simulink model "powersupply_1jan_old_top"  (R2015b)
settings: Solver=ode45  StartTime=0.0  StopTime=20*T_mach  MaxStep=4e-7  MinStep=1e-8  RelTol=1e-3
values from neighbouring files (symbols this model uses):
  c2_val = (1-V_ref/Vd_val)/(8*v2_ripple*l2_val*f_sw^2)    (= 0.0001)    [PowerSupplyScript.m]    (also in master_conv.m; master_conv2.m = 6.25e-07; matlab.mat = 1e-05; normal_buck_comparison.m = 1e-05)
  Cs = (Cs_min + Cs_max) / 2    (= 1.43223295455e-05)    [PowerSupplyScript.m]    (also in QdSnubber.m = (Cs_min + Cs_max) / 2; master_conv2.m = 3.126125e-05; matlab.mat = 2.98407954545e-05)
  delay_load = t1    (= 6e-06)    [PowerSupplyScript.m]    (also in master_conv.m; master_conv2.m; matlab.mat)
  delayVC = 2e-3    (= 0.002)    [PowerSupplyScript.m]    (also in master_conv.m = 0.001; master_conv2.m = 0; matlab.mat = 0)
  den_c1 =     [matlab.mat]
  den_c2 =     [matlab.mat]
  duty_inv = 100 - duty    (= 90)    [PowerSupplyScript.m]    (also in master_conv.m; master_conv2.m; matlab.mat)
  duty_load = (t2-t1)/T_mach*100    (= 7)    [PowerSupplyScript.m]    (also in master_conv.m; master_conv2.m; matlab.mat)
  f_sw = 50e3    (= 50000)    [PowerSupplyScript.m]    (also in master_conv.m; master_conv2.m; matlab.mat)
  frq_dc = 50    [master_conv2.m]    (also in matlab.mat = 10)
  I_ref = 10    [PowerSupplyScript.m]    (also in master_conv.m; master_conv2.m; matlab.mat)
  l1_val = Vo1*(Vd_val-Vo1)/(delta_i1*f_sw*Vd_val)    (= 0.00181818181818)    [PowerSupplyScript.m]    (also in master_conv.m = 0.000181818181818; master_conv2.m; matlab.mat; poles_locus.m = l1_val_bak)
  l2_val = 2.5*r_val*(Vd_val-V_ref)/(f_sw*Vd_val)    (= 1.36363636364e-05)    [PowerSupplyScript.m]    (also in master_conv.m; master_conv2.m = 0.00218181818182; matlab.mat = 0.002; poles_locus.m = l2_val_bak)
  num_c1 =     [matlab.mat]
  num_c2 =     [matlab.mat]
  r_val = 1    [PowerSupplyScript.m]    (also in master_conv.m; master_conv2.m; matlab.mat)
  rc2_val = 0.0001    [PowerSupplyScript.m]    (also in master_conv.m; master_conv2.m; matlab.mat)
  rl1_val = 0.0002    [PowerSupplyScript.m]    (also in master_conv.m; master_conv2.m; matlab.mat)
  rl2_val = 0.0001    [PowerSupplyScript.m]    (also in master_conv.m; master_conv2.m; matlab.mat)
  Rs = V_ref / I_ref    (= 8)    [PowerSupplyScript.m]    (also in QdSnubber.m = V_ref / I_ref; master_conv2.m; matlab.mat)
  t2 = duty * T_mach / 100    (= 2e-05)    [PowerSupplyScript.m]    (also in master_conv.m; master_conv2.m; matlab.mat)
  T_mach = 200e-6    (= 0.0002)    [PowerSupplyScript.m]    (also in master_conv.m; master_conv2.m; matlab.mat)
  V_ref = 80    [PowerSupplyScript.m]    (also in master_conv.m; master_conv2.m; matlab.mat)
  Vd_val = 110    [PowerSupplyScript.m]    (also in master_conv.m; master_conv2.m; matlab.mat)
libraries: powerlib x86, simulink x10, powerlib_meascontrol x8, simulink_extras x6
(part 1 of 2)
settings Model: Creator=Akshay  LastModifiedBy=Akshay
settings SolverCC: ZeroCrossAlgorithm=Adaptive
settings DataIOCC: SaveFormat=StructureWithTime
settings HardwareCC: ProdWordSize=32  ProdHWDeviceType=Specified

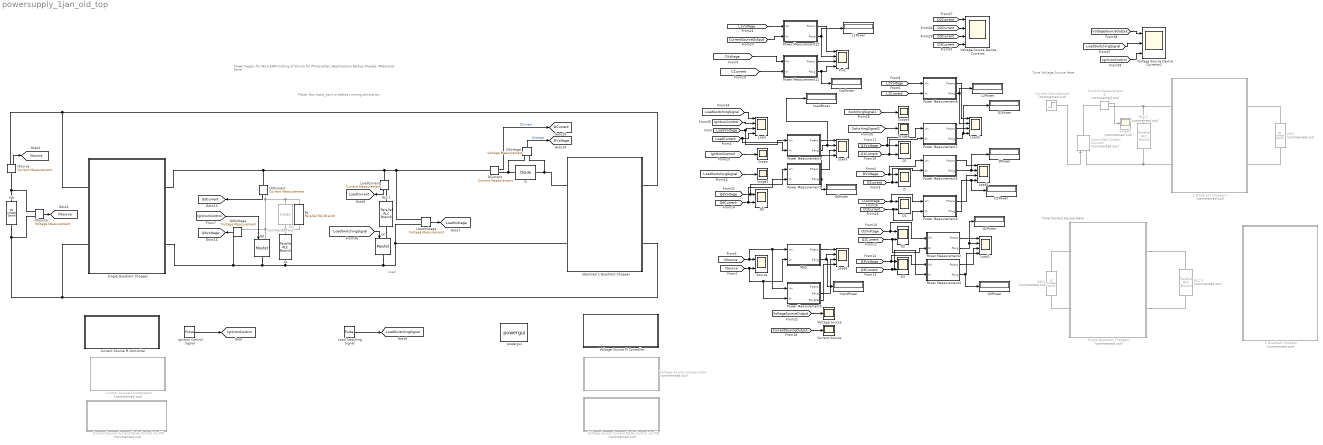
== system powersupply_1jan_old_top ==
  note: Tune Current Source Here
  note: Tune Voltage Source Here
  note: Power Supply for Wire EDM Cutting of Silicon for Photovoltaic Applications
      |
      | Akshay Khadse, Makarand Kane
  note: Load
  note: *Note: Run mast_conv.m before running simulation
  " RLC 1" : powerlib/Elements/Parallel RLC Branch  LConnTagsString=a  RConnTagsString=__new0  BranchType=R  Resistance=r_val  Inductance=1e-3  SetiL0=off  InitialCurrent=0  Capacitance=0.1e-6  Setx0=off  InitialVoltage=0  Measurements=None
  " RLC 2" : powerlib/Elements/Parallel RLC Branch  Commented=on  LConnTagsString=a  RConnTagsString=__new0  BranchType=R  Resistance=r_val  Inductance=1e-3  SetiL0=off  InitialCurrent=0  Capacitance=0.1e-6  Setx0=off  InitialVoltage=0  Measurements=None
  " RLC 3" : powerlib/Elements/Parallel RLC Branch  Commented=on  LConnTagsString=a  RConnTagsString=__new0  BranchType=R  Resistance=r_val  Inductance=1e-3  SetiL0=off  InitialCurrent=0  Capacitance=0.1e-6  Setx0=off  InitialVoltage=0  Measurements=None
  " Rs" : powerlib/Elements/Parallel RLC Branch  LConnTagsString=a  RConnTagsString=__new0  BranchType=R  Resistance=Rs  Inductance=1e-3  SetiL0=off  InitialCurrent=0  Capacitance=0.1e-6  Setx0=off  InitialVoltage=0  Measurements=None
  2 Quadrant Chopper : Subsystem  Commented=on
  2 Quadrant Chopper1 : Subsystem  Commented=on
  CapPower : Display
  Controlled Current Source1 : powerlib/Electrical Sources/Controlled Current Source  Commented=on  Initialize=on  Source_Type=AC  Amplitude=0  Phase=0  Frequency=0  Measurements=None
  Cs : powerlib/Elements/Parallel RLC Branch  LConnTagsString=a  RConnTagsString=__new0  BranchType=C  Resistance=r_val  Inductance=1e-3  SetiL0=off  InitialCurrent=0  Capacitance=Cs  Setx0=off  InitialVoltage=0  Measurements=None
  Current Disturbance1 : Step  Commented=on  Time=1e-3  After=10  SampleTime=0
  Current Measurement3 : powerlib/Measurements/Current Measurement  Commented=on  PhasorSimulation=off  OutputType=Complex  PSBequivalent=0
  Current Source : Scope
  Current Source Compensator : Subsystem  Commented=on
  Current Source Current Mode Control via PID : Subsystem  Commented=on
  Current Source PI Controller : Subsystem
  D : powerlib/Power Electronics/Diode  Ron=0.001  Lon=0  Vf=0.8  IC=0  UseSnubber=off  Rs=500  Cs=250e-9  Measurements=off
  "D " : Scope  NumInputPorts=2
  D1 : Scope  NumInputPorts=2
  D1Power : Display
  DCurrent : powerlib/Measurements/Current Measurement  PhasorSimulation=off  OutputType=Complex  PSBequivalent=0
  DPower : Display
  DVoltage : powerlib/Measurements/Voltage Measurement  PhasorSimulation=off  OutputType=Complex  PSBequivalent=0
  Ds : powerlib/Power Electronics/Diode  Commented=on  Ron=0.001  Lon=0  Vf=0.8  IC=0  UseSnubber=off  Rs=500  Cs=250e-9  Measurements=off
  ISource : powerlib/Measurements/Current Measurement  PhasorSimulation=off  OutputType=Complex  PSBequivalent=0
  Idealized 2 Quadrant Chopper : Subsystem
  Ignition Control Signal : DiscretePulseGenerator  PulseType=Time based  Period=T_mach  PulseWidth=duty_inv  PhaseDelay=t2 + delayVC
  InputPower : Display
  L1Power : Display
  L2Power : Display
  Load{,1..3,5..6} (6 alike) : Scope  NumInputPorts=4
  Load Switching Signal : DiscretePulseGenerator  PulseType=Time based  Period=T_mach  PulseWidth=duty_load  PhaseDelay=delay_load + delayVC
  LoadCurrent : powerlib/Measurements/Current Measurement  PhasorSimulation=off  OutputType=Complex  PSBequivalent=0
  LoadPower : Display
  LoadVoltage : powerlib/Measurements/Voltage Measurement  PhasorSimulation=off  OutputType=Complex  PSBequivalent=0
  PM0 : Subsystem
  Pm1 : Scope  NumInputPorts=4
  Power Measurement1 : Subsystem
  Power Measurement11 : Subsystem
  Power Measurement12 : Subsystem
  Power Measurement2 : Subsystem
  Power Measurement3 : Subsystem
  Power Measurement4 : Subsystem
  Power Measurement5 : Subsystem
  Power Measurement6 : Subsystem
  Power Measurement7 : Subsystem
  Power Measurement8 : Subsystem
  Power Measurement9 : Subsystem
  "Q1 " : Scope  NumInputPorts=2
  Q1Power : Display
  "Q2 " : Scope  NumInputPorts=2
  Q2Power : Display
  "Q3 " : Scope  NumInputPorts=2
  Q3Power : Display
  Qd : powerlib/Power Electronics/Mosfet  Ron=0.1  Lon=0  Rd=0.01  Vfd=0  IC=0  Rs=1e5  Cs=inf  Measurements=off
  "Qd " : Scope  NumInputPorts=2
  QdCurrent : powerlib/Measurements/Current Measurement  PhasorSimulation=off  OutputType=Complex  PSBequivalent=0
  QdPower : Display
  QdVoltage : powerlib/Measurements/Voltage Measurement  PhasorSimulation=off  OutputType=Complex  PSBequivalent=0
  Ql : powerlib/Power Electronics/Mosfet  Ron=0.1  Lon=0  Rd=0.01  Vfd=0  IC=0  Rs=1e5  Cs=inf  Measurements=off
  Scope{,1,5..6} (4 alike) : Scope
  Scope2 : Scope  Commented=on
  Single Quadrant Chopper : Subsystem
  Single Quadrant Chopper1 : Subsystem  Commented=on
  Source : Scope  NumInputPorts=2
  VSource : powerlib/Measurements/Voltage Measurement  PhasorSimulation=off  OutputType=Complex  PSBequivalent=0
  Vdc : powerlib/Electrical Sources/DC Voltage Source  Amplitude=Vd_val  Measurements=Voltage
  Vdc1 : powerlib/Electrical Sources/DC Voltage Source  Commented=on  Amplitude=Vd_val  Measurements=Voltage
  Vdc2 : powerlib/Electrical Sources/DC Voltage Source  Commented=on  Amplitude=Vd_val  Measurements=Voltage
  Voltage Source : Scope
  Voltage Source Device Currents : Scope  NumInputPorts=4
  Voltage Source Device Currents1 : Scope  NumInputPorts=3
  Voltage Source Compensator : Subsystem  Commented=on
  Voltage Source Current Mode Control via PID : Subsystem  Commented=on
  Voltage Source PI Controller : Subsystem
  powergui : powerlib/powergui  Priority=1  SimulationMode=Discrete  SolverType=Backward Euler  SampleTime=0.01/f_sw  frequency=60  SPID=on  DisableSnubberDevices=off  DisableRonSwitches=off  DisableVfSwitches=off  SwTol=0  DisplayEquations=off  Interpol=off  ExternalGateDelay=off  methode=off  Ts=0  FunctionMessages=off  echomessages=off  HookPort=off  EnableUseOfTLC=off  x0status=zero  frequencyindice=0  Pbase=100e6  ErrMax=1e-4  Iterations=50  UnitsV=kV  UnitsW=MW  buscounter=0  RestoreLinks=warning  ResistiveCurrentMeasurement=off  Frange=[0:2:500]  Ylog=off  Xlog=on  ShowGrid=off  save=off  variable=ZData  structure=ScopeData  ZoomFFT=off  StartTime=0.0  cycles=5  DisplayStyle=2  fundamental=50  FreqAxis=off  MaxFrequency=50000  frequencyindicesteady=1  RmsSteady=1  display=off
  tag scope: DCurrent=global, DVoltage=global, ISource=global, IgnitionControl=global, LoadCurrent=global, LoadSwitchingSignal=global, LoadVoltage=global, QdCurrent=global, QdVoltage=global, VSource=global
  wires:
  Ignition Control Signal/1 -> [IgnitionControl]
  Load Switching Signal/1 -> [LoadSwitchingSignal]
  [Q2Voltage] -> Power Measurement2/1(Vin), "Q2 "/1
  [Q2Current] -> Power Measurement2/2(Iin), "Q2 "/2
  [Q3Voltage] -> Power Measurement4/1(Vin), "Q3 "/1
  [Q3Current] -> Power Measurement4/2(Iin), "Q3 "/2
  [Q1Voltage] -> Power Measurement7/1(Vin), "Q1 "/1
  [Q1Current] -> Power Measurement7/2(Iin), "Q1 "/2
  [QdVoltage] -> Power Measurement1/1(Vin), "Qd "/1
  [QdCurrent] -> Power Measurement1/2(Iin), "Qd "/2
  [IgnitionControl] -> Scope/1
  [LoadSwitchingSignal] -> Scope1/1
  LoadCurrent/1 -> [LoadCurrent]
  LoadVoltage/1 -> [LoadVoltage]
  [IgnitionControl] -> Qd/1
  QdCurrent/1 -> [QdCurrent]
  QdVoltage/1 -> [QdVoltage]
  DVoltage/1 -> [DVoltage]  "DVoltage"
  DCurrent/1 -> [DCurrent]  "DCurrent"
  [LoadSwitchingSignal] -> Load/1
  [IgnitionControl] -> Load/2
  [LoadVoltage] -> Power Measurement9/1(Vin), Load/3
  [LoadCurrent] -> Power Measurement9/2(Iin), Load/4
  [LoadSwitchingSignal] -> Ql/1
  [SwitchingSignal2] -> Scope6/1
  [SwitchingSignal1] -> Scope5/1
  [DVoltage] -> Power Measurement5/1(Vin), "D "/1
  [DCurrent] -> Power Measurement5/2(Iin), "D "/2
  VSource/1 -> [VSource]
  ISource/1 -> [ISource]
  [VSource] -> Power Measurement3/1(Vin), PM0/1(Vin), Source/1
  [ISource] -> Power Measurement3/2(Iin), PM0/2(Iin), Source/2
  [D1Voltage] -> Power Measurement6/1(Vin), D1/1
  Current Disturbance1/1 -> Controlled Current Source1/1
  Current Measurement3/1 -> Scope2/1
  Power Measurement2/1(Ptrans) -> Load1/1
  Power Measurement2/2(Pavg) -> Load1/2, Q2Power/1
  Power Measurement4/1(Ptrans) -> Load1/3
  Power Measurement4/2(Pavg) -> Load1/4, Q3Power/1
  [D1Current] -> Power Measurement6/2(Iin), D1/2
  Power Measurement5/1(Ptrans) -> Load5/1
  Power Measurement5/2(Pavg) -> Load5/2, DPower/1
  Power Measurement6/1(Ptrans) -> Load5/3
  Power Measurement6/2(Pavg) -> Load5/4, D1Power/1
  Power Measurement9/1(Ptrans) -> Load3/1
  Power Measurement9/2(Pavg) -> Load3/2, LoadPower/1
  Power Measurement1/1(Ptrans) -> Load3/3
  Power Measurement1/2(Pavg) -> Load3/4, QdPower/1
  PM0/1(Ptrans) -> Load6/1
  PM0/2(Pavg) -> Load6/2, InputPower/1
  [L2Current] -> Power Measurement8/2(Iin)
  [L2Voltage] -> Power Measurement8/1(Vin)
  Power Measurement7/2(Pavg) -> Load2/4, Q1Power/1
  Power Measurement7/1(Ptrans) -> Load2/3
  Power Measurement8/1(Ptrans) -> Load2/1
  Power Measurement8/2(Pavg) -> Load2/2, L2Power/1
  [CVoltage] -> Power Measurement11/1(Vin)
  [CCurrent] -> Power Measurement11/2(Iin)
  Power Measurement11/1(Ptrans) -> Pm1/3
  Power Measurement11/2(Pavg) -> CapPower/1, Pm1/4
  [L1Voltage] -> Power Measurement12/1(Vin)
  [CurrentSourceOutput] -> Power Measurement12/2(Iin)
  Power Measurement12/1(Ptrans) -> Pm1/1
  Power Measurement12/2(Pavg) -> L1Power/1, Pm1/2
  [VoltageSourceOutput] -> Voltage Source/1
  [CurrentSourceOutput] -> Current Source/1
  Power Measurement3/2(Pavg) -> Load6/3
  Power Measurement3/3(PavgFB) -> Load6/4
  [Q2Current] -> Voltage Source Device Currents/1
  [Q3Current] -> Voltage Source Device Currents/3
  [D3Current] -> Voltage Source Device Currents/4
  [D2Current] -> Voltage Source Device Currents/2
  [VoltageSourceOutput] -> Voltage Source Device Currents1/1
  [LoadSwitchingSignal] -> Voltage Source Device Currents1/2
  [IgnitionControl] -> Voltage Source Device Currents1/3
  connections:
  LoadCurrent/RConn1 -- " RLC 1"/LConn1
  Ds/LConn1 -- QdVoltage/LConn2 -- Qd/LConn1 -- QdCurrent/RConn1 -- " Rs"/LConn1
  DVoltage/LConn1 -- DCurrent/RConn1 -- D/LConn1
  DCurrent/LConn1 -- LoadVoltage/LConn1 -- Single Quadrant Chopper/RConn1 -- QdCurrent/LConn1 -- LoadCurrent/LConn1
  Idealized 2 Quadrant Chopper/RConn1 -- ISource/RConn1 -- Single Quadrant Chopper/LConn1
  Idealized 2 Quadrant Chopper/RConn2 -- VSource/LConn2 -- Vdc/LConn1 -- Single Quadrant Chopper/LConn2
  Ql/LConn1 -- " RLC 1"/RConn1
  Qd/RConn1 -- Idealized 2 Quadrant Chopper/LConn2 -- LoadVoltage/LConn2 -- Ql/RConn1 -- Cs/RConn1 -- Single Quadrant Chopper/RConn2 -- QdVoltage/LConn1
  ISource/LConn1 -- Vdc/RConn1 -- VSource/LConn1
  " RLC 2"/LConn1 -- Current Measurement3/RConn1 -- 2 Quadrant Chopper1/LConn1
  " RLC 2"/RConn1 -- Controlled Current Source1/LConn1 -- 2 Quadrant Chopper1/LConn2
  Vdc1/RConn1 -- 2 Quadrant Chopper1/RConn1
  Vdc1/LConn1 -- 2 Quadrant Chopper1/RConn2
  Vdc2/RConn1 -- Single Quadrant Chopper1/LConn1
  Vdc2/LConn1 -- Single Quadrant Chopper1/LConn2
  Single Quadrant Chopper1/RConn1 -- " RLC 3"/LConn1
  Single Quadrant Chopper1/RConn2 -- " RLC 3"/RConn1
  Ds/RConn1 -- " Rs"/RConn1 -- Cs/LConn1
  Controlled Current Source1/RConn1 -- Current Measurement3/LConn1
  Idealized 2 Quadrant Chopper/LConn1 -- DVoltage/LConn2 -- D/RConn1

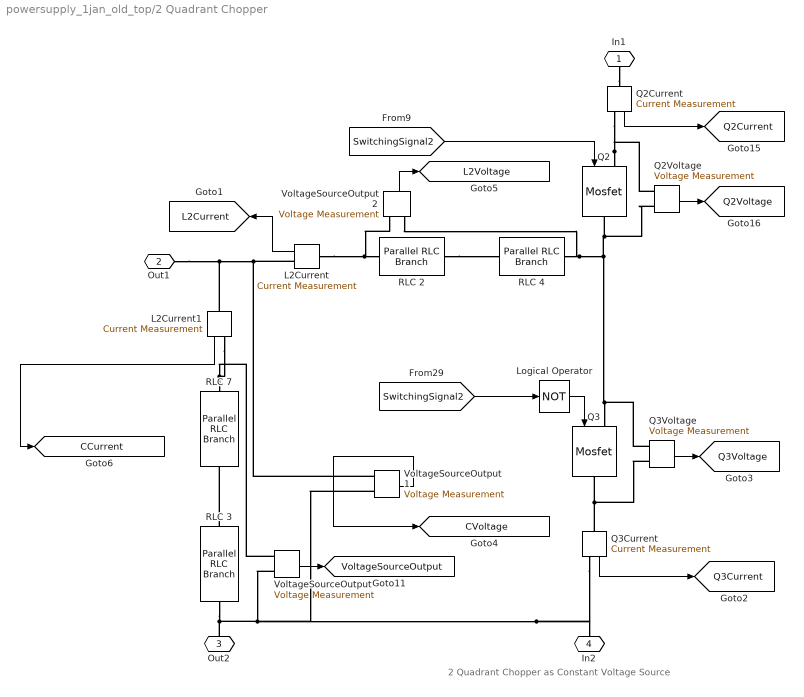
== system powersupply_1jan_old_top/2 Quadrant Chopper ==
  note: 2 Quadrant Chopper as Constant Voltage Source
  " RLC 2" : powerlib/Elements/Parallel RLC Branch  LConnTagsString=a  RConnTagsString=__new0  BranchType=R  Resistance=rl2_val  Inductance=5e-6  SetiL0=off  InitialCurrent=0  Capacitance=0.3e-6  Setx0=off  InitialVoltage=0  Measurements=None
  " RLC 3" : powerlib/Elements/Parallel RLC Branch  LConnTagsString=a  RConnTagsString=__new0  BranchType=C  Resistance=1  Inductance=1e-3  SetiL0=off  InitialCurrent=0  Capacitance=c2_val  Setx0=off  InitialVoltage=50  Measurements=None
  " RLC 4" : powerlib/Elements/Parallel RLC Branch  LConnTagsString=a  RConnTagsString=__new0  BranchType=L  Resistance=50  Inductance=l2_val  SetiL0=off  InitialCurrent=0  Capacitance=0.3e-6  Setx0=off  InitialVoltage=0  Measurements=None
  " RLC 7" : powerlib/Elements/Parallel RLC Branch  LConnTagsString=a  RConnTagsString=__new0  BranchType=R  Resistance=rc2_val  Inductance=1e-3  SetiL0=off  InitialCurrent=0  Capacitance=0.1e-6  Setx0=off  InitialVoltage=0  Measurements=None
  L2Current : powerlib/Measurements/Current Measurement  PhasorSimulation=off  OutputType=Complex  PSBequivalent=0
  L2Current1 : powerlib/Measurements/Current Measurement  PhasorSimulation=off  OutputType=Complex  PSBequivalent=0
  Logical Operator : Logic  Operator=NOT  AllPortsSameDT=off  OutDataTypeStr=boolean
  Q2 : powerlib/Power Electronics/Mosfet  Ron=0.1  Lon=0  Rd=0.01  Vfd=0  IC=0  Rs=1e5  Cs=inf  Measurements=off
  Q2Current : powerlib/Measurements/Current Measurement  PhasorSimulation=off  OutputType=Complex  PSBequivalent=0
  Q2Voltage : powerlib/Measurements/Voltage Measurement  PhasorSimulation=off  OutputType=Complex  PSBequivalent=0
  Q3 : powerlib/Power Electronics/Mosfet  Ron=0.1  Lon=0  Rd=0.01  Vfd=0  IC=0  Rs=1e5  Cs=inf  Measurements=off
  Q3Current : powerlib/Measurements/Current Measurement  PhasorSimulation=off  OutputType=Complex  PSBequivalent=0
  Q3Voltage : powerlib/Measurements/Voltage Measurement  PhasorSimulation=off  OutputType=Complex  PSBequivalent=0
  VoltageSourceOutput : powerlib/Measurements/Voltage Measurement  PhasorSimulation=off  OutputType=Complex  PSBequivalent=0
  VoltageSourceOutput1 : powerlib/Measurements/Voltage Measurement  PhasorSimulation=off  OutputType=Complex  PSBequivalent=0
  VoltageSourceOutput2 : powerlib/Measurements/Voltage Measurement  PhasorSimulation=off  OutputType=Complex  PSBequivalent=0
  In1 : PMIOPort  Port=1  Side=Right
  Out1 : PMIOPort  Port=2  Side=Left
  Out2 : PMIOPort  Port=3  Side=Left
  In2 : PMIOPort  Port=4  Side=Right
  tag scope: CCurrent=global, CVoltage=global, L2Current=global, L2Voltage=global, Q2Current=global, Q2Voltage=global, Q3Current=global, Q3Voltage=global, VoltageSourceOutput=global
  wires:
  Logical Operator/1 -> Q3/1
  VoltageSourceOutput/1 -> [VoltageSourceOutput]
  Q3Current/1 -> [Q3Current]
  Q3Voltage/1 -> [Q3Voltage]
  Q2Voltage/1 -> [Q2Voltage]
  Q2Current/1 -> [Q2Current]
  [SwitchingSignal2] -> Q2/1
  [SwitchingSignal2] -> Logical Operator/1
  L2Current/1 -> [L2Current]
  VoltageSourceOutput1/1 -> [CVoltage]
  VoltageSourceOutput2/1 -> [L2Voltage]
  L2Current1/1 -> [CCurrent]
  connections:
  " RLC 3"/RConn1 -- VoltageSourceOutput1/LConn2 -- Q3Current/RConn1 -- In2/RConn1 -- VoltageSourceOutput/LConn2 -- Out2/RConn1
  " RLC 3"/LConn1 -- " RLC 7"/RConn1
  Q3Voltage/LConn2 -- Q3Current/LConn1 -- Q3/RConn1
  Q2/LConn1 -- Q2Voltage/LConn1 -- Q2Current/RConn1
  " RLC 2"/RConn1 -- " RLC 4"/LConn1
  In1/RConn1 -- Q2Current/LConn1
  Out1/RConn1 -- L2Current1/LConn1 -- VoltageSourceOutput1/LConn1 -- L2Current/RConn1
  " RLC 4"/RConn1 -- Q3Voltage/LConn1 -- Q3/LConn1 -- Q2Voltage/LConn2 -- Q2/RConn1 -- VoltageSourceOutput2/LConn2
  L2Current/LConn1 -- VoltageSourceOutput2/LConn1 -- " RLC 2"/LConn1
  " RLC 7"/LConn1 -- L2Current1/RConn1 -- VoltageSourceOutput/LConn1

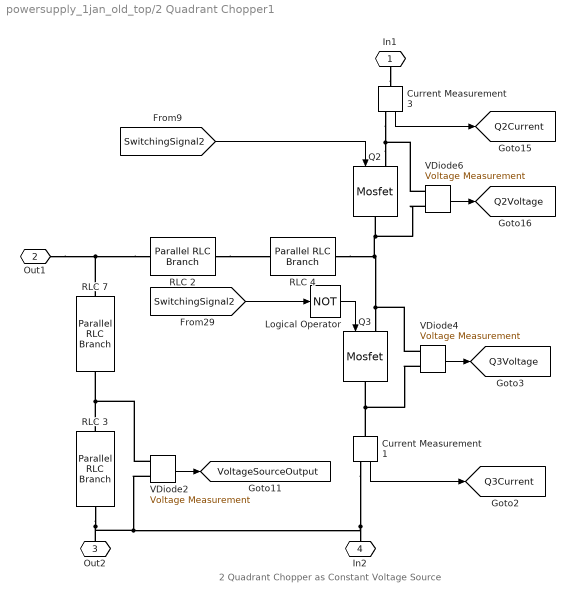
== system powersupply_1jan_old_top/2 Quadrant Chopper1 ==
  note: 2 Quadrant Chopper as Constant Voltage Source
  " RLC 2" : powerlib/Elements/Parallel RLC Branch  LConnTagsString=a  RConnTagsString=__new0  BranchType=R  Resistance=rl2_val  Inductance=5e-6  SetiL0=off  InitialCurrent=0  Capacitance=0.3e-6  Setx0=off  InitialVoltage=0  Measurements=None
  " RLC 3" : powerlib/Elements/Parallel RLC Branch  LConnTagsString=a  RConnTagsString=__new0  BranchType=C  Resistance=1  Inductance=1e-3  SetiL0=off  InitialCurrent=0  Capacitance=c2_val  Setx0=off  InitialVoltage=50  Measurements=None
  " RLC 4" : powerlib/Elements/Parallel RLC Branch  LConnTagsString=a  RConnTagsString=__new0  BranchType=L  Resistance=50  Inductance=l2_val  SetiL0=off  InitialCurrent=0  Capacitance=0.3e-6  Setx0=off  InitialVoltage=0  Measurements=None
  " RLC 7" : powerlib/Elements/Parallel RLC Branch  LConnTagsString=a  RConnTagsString=__new0  BranchType=R  Resistance=rc2_val  Inductance=1e-3  SetiL0=off  InitialCurrent=0  Capacitance=0.1e-6  Setx0=off  InitialVoltage=0  Measurements=None
  Current Measurement1 : powerlib/Measurements/Current Measurement  PhasorSimulation=off  OutputType=Complex  PSBequivalent=0
  Current Measurement3 : powerlib/Measurements/Current Measurement  PhasorSimulation=off  OutputType=Complex  PSBequivalent=0
  Logical Operator : Logic  Operator=NOT  AllPortsSameDT=off  OutDataTypeStr=boolean
  Q2 : powerlib/Power Electronics/Mosfet  Ron=0.1  Lon=0  Rd=0.01  Vfd=0  IC=0  Rs=1e5  Cs=inf  Measurements=off
  Q3 : powerlib/Power Electronics/Mosfet  Ron=0.1  Lon=0  Rd=0.01  Vfd=0  IC=0  Rs=1e5  Cs=inf  Measurements=off
  VDiode2 : powerlib/Measurements/Voltage Measurement  PhasorSimulation=off  OutputType=Complex  PSBequivalent=0
  VDiode4 : powerlib/Measurements/Voltage Measurement  PhasorSimulation=off  OutputType=Complex  PSBequivalent=0
  VDiode6 : powerlib/Measurements/Voltage Measurement  PhasorSimulation=off  OutputType=Complex  PSBequivalent=0
  In1 : PMIOPort  Port=1  Side=Right
  Out1 : PMIOPort  Port=2  Side=Left
  Out2 : PMIOPort  Port=3  Side=Left
  In2 : PMIOPort  Port=4  Side=Right
  tag scope: Q2Current=global, Q2Voltage=global, Q3Current=global, Q3Voltage=global, VoltageSourceOutput=global
  wires:
  Logical Operator/1 -> Q3/1
  VDiode2/1 -> [VoltageSourceOutput]
  Current Measurement1/1 -> [Q3Current]
  VDiode4/1 -> [Q3Voltage]
  VDiode6/1 -> [Q2Voltage]
  Current Measurement3/1 -> [Q2Current]
  [SwitchingSignal2] -> Q2/1
  [SwitchingSignal2] -> Logical Operator/1
  connections:
  " RLC 3"/RConn1 -- Current Measurement1/RConn1 -- In2/RConn1 -- VDiode2/LConn2 -- Out2/RConn1
  VDiode2/LConn1 -- " RLC 3"/LConn1 -- " RLC 7"/RConn1
  VDiode4/LConn2 -- Current Measurement1/LConn1 -- Q3/RConn1
  Q2/LConn1 -- VDiode6/LConn1 -- Current Measurement3/RConn1
  " RLC 2"/RConn1 -- " RLC 4"/LConn1
  In1/RConn1 -- Current Measurement3/LConn1
  " RLC 2"/LConn1 -- " RLC 7"/LConn1 -- Out1/RConn1
  " RLC 4"/RConn1 -- VDiode4/LConn1 -- Q3/LConn1 -- VDiode6/LConn2 -- Q2/RConn1

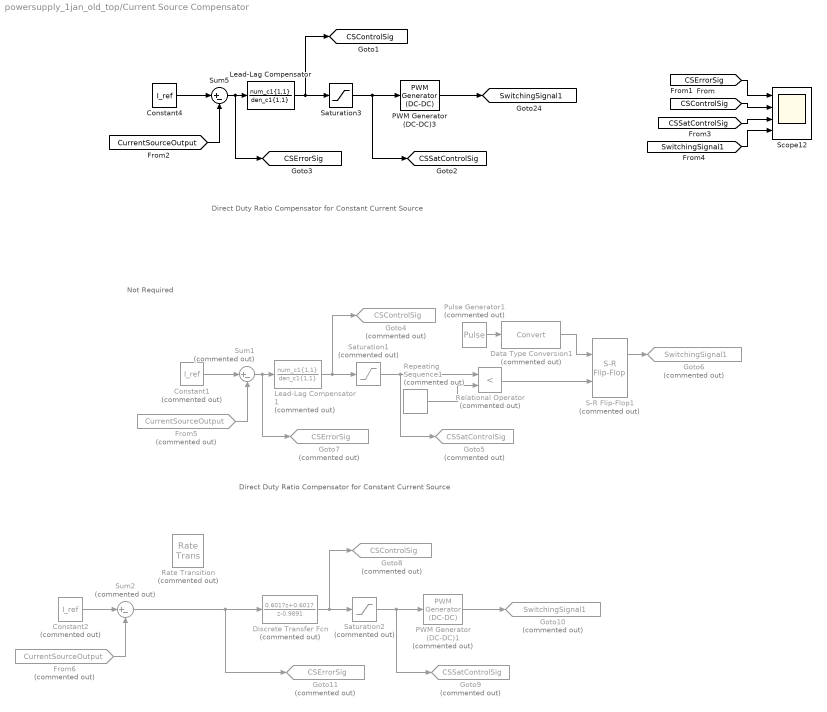
== system powersupply_1jan_old_top/Current Source Compensator ==
  note: Not Required
  note: Direct Duty Ratio Compensator for Constant Current Source
  note: Direct Duty Ratio Compensator for Constant Current Source
  Constant1 : Constant  Commented=on  Value=I_ref
  Constant2 : Constant  Commented=on  Value=I_ref
  Constant4 : Constant  Value=I_ref
  Data Type Conversion1 : DataTypeConversion  Commented=on
  Discrete Transfer Fcn : DiscreteTransferFcn  Commented=on  Numerator=[0.6017 0.6017]  Denominator=[1 -0.9891]
  From5 : From  Commented=on  GotoTag=CurrentSourceOutput  TagVisibility=global
  From6 : From  Commented=on  GotoTag=CurrentSourceOutput  TagVisibility=global
  Goto10 : Goto  Commented=on  GotoTag=SwitchingSignal1  TagVisibility=global
  Goto11 : Goto  Commented=on  GotoTag=CSErrorSig  TagVisibility=global
  Goto4 : Goto  Commented=on  GotoTag=CSControlSig  TagVisibility=global
  Goto5 : Goto  Commented=on  GotoTag=CSSatControlSig  TagVisibility=global
  Goto6 : Goto  Commented=on  GotoTag=SwitchingSignal1  TagVisibility=global
  Goto7 : Goto  Commented=on  GotoTag=CSErrorSig  TagVisibility=global
  Goto8 : Goto  Commented=on  GotoTag=CSControlSig  TagVisibility=global
  Goto9 : Goto  Commented=on  GotoTag=CSSatControlSig  TagVisibility=global
  Lead-Lag Compensator : TransferFcn  Numerator=num_c1{1,1}  Denominator=den_c1{1,1}
  Lead-Lag Compensator1 : TransferFcn  Commented=on  Numerator=num_c1{1,1}  Denominator=den_c1{1,1}
  PWM Generator (DC-DC)1 : powerlib_meascontrol/Pulse & Signal Generators/PWM Generator (DC-DC)  Commented=on  Fsw=f_sw  Ts=0
  PWM Generator (DC-DC)3 : powerlib_meascontrol/Pulse & Signal Generators/PWM Generator (DC-DC)  Fsw=f_sw  Ts=0
  Pulse Generator1 : DiscretePulseGenerator  Commented=on  PulseType=Time based  Period=1/f_sw  PulseWidth=5
  Rate Transition : RateTransition  Commented=on  OutPortSampleTime=0.01/f_sw
  Relational Operator : RelationalOperator  Commented=on  Operator=<  OutDataTypeStr=boolean
  Repeating Sequence1 : simulink/Sources/Repeating Sequence  Commented=on  rep_seq_t=[0 1/f_sw]  rep_seq_y=[0 1]
  S-R Flip-Flop1 : simulink_extras/Flip Flops/S-R Flip-Flop  Commented=on  initial_condition=0
  Saturation1 : Saturate  Commented=on  UpperLimit=0.99  LowerLimit=0
  Saturation2 : Saturate  Commented=on  UpperLimit=0.99  LowerLimit=0
  Saturation3 : Saturate  UpperLimit=0.99  LowerLimit=0
  Scope12 : Scope  NumInputPorts=4
  Sum1 : Sum  Commented=on  Inputs=|+-
  Sum2 : Sum  Commented=on  Inputs=|+-
  Sum5 : Sum  Inputs=|+-
  tag scope: CSControlSig=global, CSErrorSig=global, CSSatControlSig=global, SwitchingSignal1=global
  wires:
  Sum5/1 -> [CSErrorSig], Lead-Lag Compensator/1
  Constant4/1 -> Sum5/1
  [CurrentSourceOutput] -> Sum5/2
  Lead-Lag Compensator/1 -> Saturation3/1, [CSControlSig]
  Saturation3/1 -> [CSSatControlSig], PWM Generator (DC-DC)3/1
  PWM Generator (DC-DC)3/1 -> [SwitchingSignal1]
  [CSErrorSig] -> Scope12/1
  [CSControlSig] -> Scope12/2
  [CSSatControlSig] -> Scope12/3
  [SwitchingSignal1] -> Scope12/4
  Sum1/1 -> Goto7/1, Lead-Lag Compensator1/1
  Constant1/1 -> Sum1/1
  From5/1 -> Sum1/2
  Lead-Lag Compensator1/1 -> Saturation1/1, Goto4/1
  Saturation1/1 -> Relational Operator/1, Goto5/1
  Repeating Sequence1/1 -> Relational Operator/2
  S-R Flip-Flop1/1 -> Goto6/1
  Pulse Generator1/1 -> Data Type Conversion1/1
  Data Type Conversion1/1 -> S-R Flip-Flop1/1
  Relational Operator/1 -> S-R Flip-Flop1/2
  Constant2/1 -> Sum2/1
  From6/1 -> Sum2/2
  Discrete Transfer Fcn/1 -> Goto8/1, Saturation2/1
  Saturation2/1 -> Goto9/1, PWM Generator (DC-DC)1/1
  PWM Generator (DC-DC)1/1 -> Goto10/1
  Sum2/1 -> Goto11/1, Discrete Transfer Fcn/1

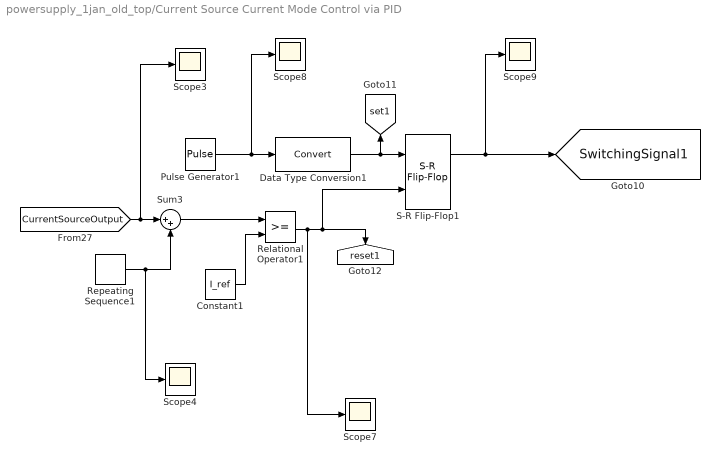
== system powersupply_1jan_old_top/Current Source Current Mode Control via PID ==
  Constant1 : Constant  Value=I_ref
  Data Type Conversion1 : DataTypeConversion
  Pulse Generator1 : DiscretePulseGenerator  PulseType=Time based  Period=1/f_sw  PulseWidth=5
  Relational Operator1 : RelationalOperator  OutDataTypeStr=boolean
  Repeating Sequence1 : simulink/Sources/Repeating Sequence  rep_seq_t=[0 1/f_sw]  rep_seq_y=[0 0]
  S-R Flip-Flop1 : simulink_extras/Flip Flops/S-R Flip-Flop  initial_condition=0
  Scope{3..4,7..9} (5 alike) : Scope
  Sum3 : Sum  Inputs=|++
  tag scope: SwitchingSignal1=global, reset1=global, set1=global
  wires:
  Pulse Generator1/1 -> Scope8/1, Data Type Conversion1/1
  Data Type Conversion1/1 -> S-R Flip-Flop1/1, [set1]
  Relational Operator1/1 -> Scope7/1, S-R Flip-Flop1/2, [reset1]
  S-R Flip-Flop1/1 -> Scope9/1, [SwitchingSignal1]
  [CurrentSourceOutput] -> Scope3/1, Sum3/1
  Repeating Sequence1/1 -> Scope4/1, Sum3/2
  Sum3/1 -> Relational Operator1/1
  Constant1/1 -> Relational Operator1/2

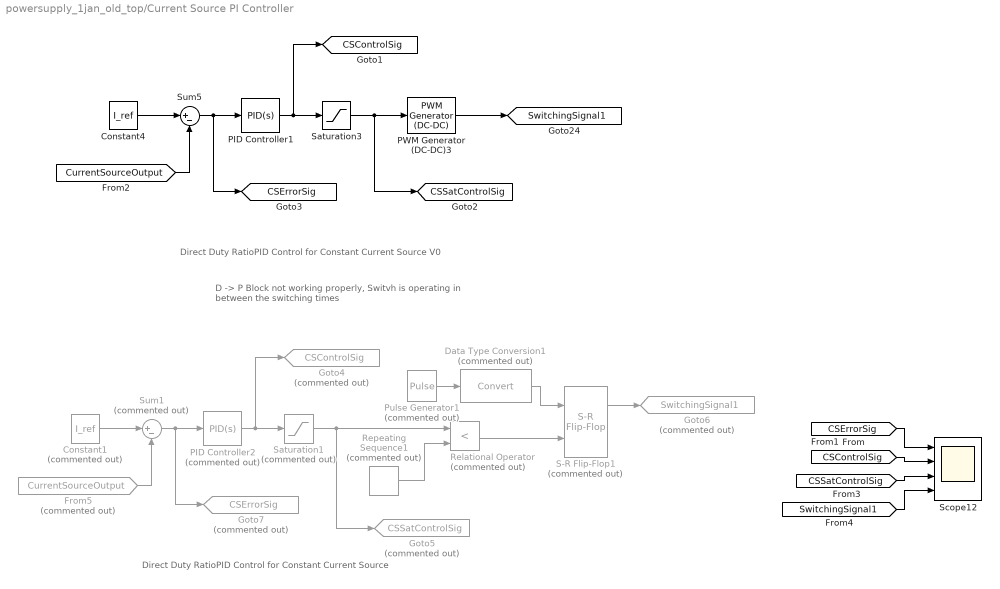
== system powersupply_1jan_old_top/Current Source PI Controller ==
  note: D -> P Block not working properly,
      | Switvh is operating in between the switching times
  note: Direct Duty RatioPID Control for Constant Current Source V0
  note: Direct Duty RatioPID Control for Constant Current Source
  Constant1 : Constant  Commented=on  Value=I_ref
  Constant4 : Constant  Value=I_ref
  Data Type Conversion1 : DataTypeConversion  Commented=on
  From5 : From  Commented=on  GotoTag=CurrentSourceOutput  TagVisibility=global
  Goto4 : Goto  Commented=on  GotoTag=CSControlSig  TagVisibility=global
  Goto5 : Goto  Commented=on  GotoTag=CSSatControlSig  TagVisibility=global
  Goto6 : Goto  Commented=on  GotoTag=SwitchingSignal1  TagVisibility=global
  Goto7 : Goto  Commented=on  GotoTag=CSErrorSig  TagVisibility=global
  PID Controller1 : simulink/Continuous/PID Controller  Controller=PID  TimeDomain=Continuous-time  SampleTime=-1  IntegratorMethod=Forward Euler  FilterMethod=Forward Euler  Form=Parallel  UseFilter=on  ControllerParametersSource=internal  P=3  I=0  D=0  N=5  InitialConditionSource=internal  InitialConditionForIntegrator=0  InitialConditionForFilter=0  ExternalReset=none  LimitOutput=off  UpperSaturationLimit=inf  LowerSaturationLimit=-inf  LinearizeAsGain=on  AntiWindupMode=none  Kb=1  TrackingMode=off  Kt=1  PParamMin=[]  PParamMax=[]  IParamMin=[]  IParamMax=[]  DParamMin=[]  DParamMax=[]  NParamMin=[]  NParamMax=[]  KbParamMin=[]  KbParamMax=[]  KtParamMin=[]  KtParamMax=[]  POutMin=[]  POutMax=[]  IOutMin=[]  IOutMax=[]  DOutMin=[]  DOutMax=[]  NOutMin=[]  NOutMax=[]  KbOutMin=[]  KbOutMax=[]  KtOutMin=[]  KtOutMax=[]  IntegratorOutMin=[]  IntegratorOutMax=[]  FilterOutMin=[]  FilterOutMax=[]  SumOutMin=[]  SumOutMax=[]  SumI1OutMin=[]  SumI1OutMax=[]  SumI2OutMin=[]  SumI2OutMax=[]  SumI3OutMin=[]  SumI3OutMax=[]  SumDOutMin=[]  SumDOutMax=[]  SaturationOutMin=[]  SaturationOutMax=[]  IntegratorContinuousStateAttributes=''  IntegratorStateMustResolveToSignalObject=off  IntegratorRTWStateStorageClass=Auto  FilterContinuousStateAttributes=''  FilterStateMustResolveToSignalObject=off  FilterRTWStateStorageClass=Auto  DifferentiatorICPrevScaledInput=0  DifferentiatorOutMin=[]  DifferentiatorOutMax=[]
  PID Controller2 : simulink/Continuous/PID Controller  Commented=on  Controller=PID  TimeDomain=Continuous-time  SampleTime=-1  IntegratorMethod=Forward Euler  FilterMethod=Forward Euler  Form=Parallel  UseFilter=on  ControllerParametersSource=internal  P=1  I=0  D=0  N=5  InitialConditionSource=internal  InitialConditionForIntegrator=0  InitialConditionForFilter=0  ExternalReset=none  LimitOutput=off  UpperSaturationLimit=inf  LowerSaturationLimit=-inf  LinearizeAsGain=on  AntiWindupMode=none  Kb=1  TrackingMode=off  Kt=1  PParamMin=[]  PParamMax=[]  IParamMin=[]  IParamMax=[]  DParamMin=[]  DParamMax=[]  NParamMin=[]  NParamMax=[]  KbParamMin=[]  KbParamMax=[]  KtParamMin=[]  KtParamMax=[]  POutMin=[]  POutMax=[]  IOutMin=[]  IOutMax=[]  DOutMin=[]  DOutMax=[]  NOutMin=[]  NOutMax=[]  KbOutMin=[]  KbOutMax=[]  KtOutMin=[]  KtOutMax=[]  IntegratorOutMin=[]  IntegratorOutMax=[]  FilterOutMin=[]  FilterOutMax=[]  SumOutMin=[]  SumOutMax=[]  SumI1OutMin=[]  SumI1OutMax=[]  SumI2OutMin=[]  SumI2OutMax=[]  SumI3OutMin=[]  SumI3OutMax=[]  SumDOutMin=[]  SumDOutMax=[]  SaturationOutMin=[]  SaturationOutMax=[]  IntegratorContinuousStateAttributes=''  IntegratorStateMustResolveToSignalObject=off  IntegratorRTWStateStorageClass=Auto  FilterContinuousStateAttributes=''  FilterStateMustResolveToSignalObject=off  FilterRTWStateStorageClass=Auto  DifferentiatorICPrevScaledInput=0  DifferentiatorOutMin=[]  DifferentiatorOutMax=[]
  PWM Generator (DC-DC)3 : powerlib_meascontrol/Pulse & Signal Generators/PWM Generator (DC-DC)  Fsw=f_sw  Ts=0
  Pulse Generator1 : DiscretePulseGenerator  Commented=on  PulseType=Time based  Period=1/f_sw  PulseWidth=5
  Relational Operator : RelationalOperator  Commented=on  Operator=<  OutDataTypeStr=boolean
  Repeating Sequence1 : simulink/Sources/Repeating Sequence  Commented=on  rep_seq_t=[0 1/f_sw]  rep_seq_y=[0 1]
  S-R Flip-Flop1 : simulink_extras/Flip Flops/S-R Flip-Flop  Commented=on  initial_condition=0
  Saturation1 : Saturate  Commented=on  UpperLimit=0.99  LowerLimit=0
  Saturation3 : Saturate  UpperLimit=0.99  LowerLimit=0
  Scope12 : Scope  NumInputPorts=4
  Sum1 : Sum  Commented=on  Inputs=|+-
  Sum5 : Sum  Inputs=|+-
  tag scope: CSControlSig=global, CSErrorSig=global, CSSatControlSig=global, SwitchingSignal1=global
  wires:
  Sum5/1 -> [CSErrorSig], PID Controller1/1
  Constant4/1 -> Sum5/1
  [CurrentSourceOutput] -> Sum5/2
  PID Controller1/1 -> Saturation3/1, [CSControlSig]
  Saturation3/1 -> [CSSatControlSig], PWM Generator (DC-DC)3/1
  PWM Generator (DC-DC)3/1 -> [SwitchingSignal1]
  [CSErrorSig] -> Scope12/1
  [CSControlSig] -> Scope12/2
  [CSSatControlSig] -> Scope12/3
  [SwitchingSignal1] -> Scope12/4
  Sum1/1 -> Goto7/1, PID Controller2/1
  Constant1/1 -> Sum1/1
  From5/1 -> Sum1/2
  PID Controller2/1 -> Saturation1/1, Goto4/1
  Repeating Sequence1/1 -> Relational Operator/2
  Relational Operator/1 -> S-R Flip-Flop1/2
  Saturation1/1 -> Relational Operator/1, Goto5/1
  S-R Flip-Flop1/1 -> Goto6/1
  Data Type Conversion1/1 -> S-R Flip-Flop1/1
  Pulse Generator1/1 -> Data Type Conversion1/1

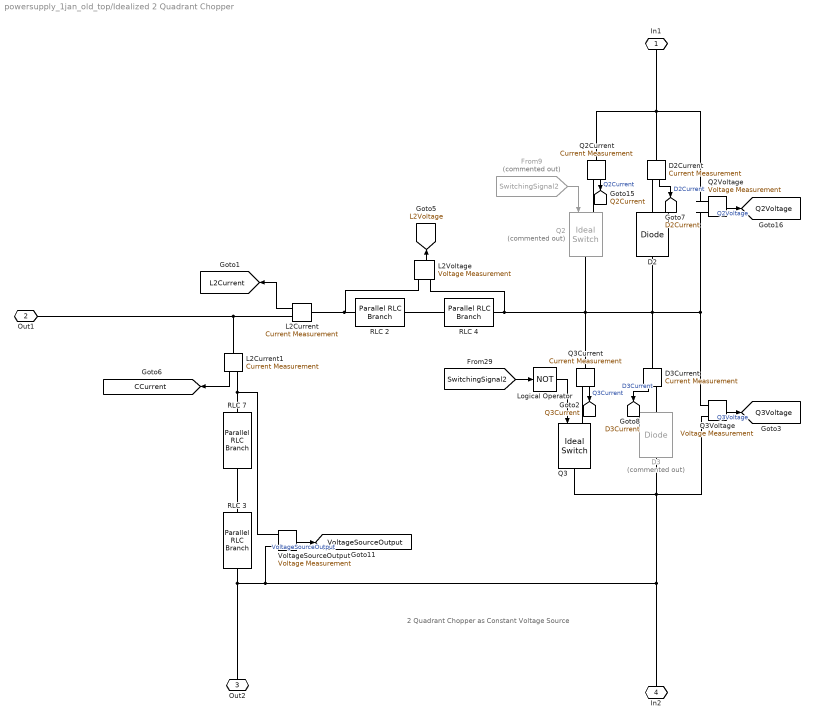
== system powersupply_1jan_old_top/Idealized 2 Quadrant Chopper ==
  note: 2 Quadrant Chopper as Constant Voltage Source
  " RLC 2" : powerlib/Elements/Parallel RLC Branch  LConnTagsString=a  RConnTagsString=__new0  BranchType=R  Resistance=rl2_val  Inductance=5e-6  SetiL0=off  InitialCurrent=0  Capacitance=0.3e-6  Setx0=off  InitialVoltage=0  Measurements=None
  " RLC 3" : powerlib/Elements/Parallel RLC Branch  LConnTagsString=a  RConnTagsString=__new0  BranchType=C  Resistance=1  Inductance=1e-3  SetiL0=off  InitialCurrent=0  Capacitance=c2_val  Setx0=off  InitialVoltage=50  Measurements=None
  " RLC 4" : powerlib/Elements/Parallel RLC Branch  LConnTagsString=a  RConnTagsString=__new0  BranchType=L  Resistance=50  Inductance=l2_val  SetiL0=off  InitialCurrent=0  Capacitance=0.3e-6  Setx0=off  InitialVoltage=0  Measurements=None
  " RLC 7" : powerlib/Elements/Parallel RLC Branch  LConnTagsString=a  RConnTagsString=__new0  BranchType=R  Resistance=rc2_val  Inductance=1e-3  SetiL0=off  InitialCurrent=0  Capacitance=0.1e-6  Setx0=off  InitialVoltage=0  Measurements=None
  D2 : powerlib/Power Electronics/Diode  Ron=0.001  Lon=0  Vf=0.8  IC=0  UseSnubber=off  Rs=inf  Cs=0  Measurements=off
  D2Current : powerlib/Measurements/Current Measurement  PhasorSimulation=off  OutputType=Complex  PSBequivalent=0
  D3 : powerlib/Power Electronics/Diode  Commented=on  Ron=0.001  Lon=0  Vf=0.8  IC=0  UseSnubber=off  Rs=inf  Cs=0  Measurements=off
  D3Current : powerlib/Measurements/Current Measurement  PhasorSimulation=off  OutputType=Complex  PSBequivalent=0
  From9 : From  Commented=on  GotoTag=SwitchingSignal2  TagVisibility=global
  L2Current : powerlib/Measurements/Current Measurement  PhasorSimulation=off  OutputType=Complex  PSBequivalent=0
  L2Current1 : powerlib/Measurements/Current Measurement  PhasorSimulation=off  OutputType=Complex  PSBequivalent=0
  L2Voltage : powerlib/Measurements/Voltage Measurement  PhasorSimulation=off  OutputType=Complex  PSBequivalent=0
  Logical Operator : Logic  Operator=NOT  AllPortsSameDT=off  OutDataTypeStr=boolean
  Q2 : powerlib/Power Electronics/Ideal Switch  Commented=on  Ron=0.001  Lon=0  IC=0  Rs=1e5  Cs=inf  Measurements=off
  Q2Current : powerlib/Measurements/Current Measurement  PhasorSimulation=off  OutputType=Complex  PSBequivalent=0
  Q2Voltage : powerlib/Measurements/Voltage Measurement  PhasorSimulation=off  OutputType=Complex  PSBequivalent=0
  Q3 : powerlib/Power Electronics/Ideal Switch  Ron=0.001  Lon=0  IC=0  Rs=1e5  Cs=inf  Measurements=off
  Q3Current : powerlib/Measurements/Current Measurement  PhasorSimulation=off  OutputType=Complex  PSBequivalent=0
  Q3Voltage : powerlib/Measurements/Voltage Measurement  PhasorSimulation=off  OutputType=Complex  PSBequivalent=0
  VoltageSourceOutput : powerlib/Measurements/Voltage Measurement  PhasorSimulation=off  OutputType=Complex  PSBequivalent=0
  In1 : PMIOPort  Port=1  Side=Right
  Out1 : PMIOPort  Port=2  Side=Left
  Out2 : PMIOPort  Port=3  Side=Left
  In2 : PMIOPort  Port=4  Side=Right
  tag scope: CCurrent=global, D2Current=global, D3Current=global, L2Current=global, L2Voltage=global, Q2Current=global, Q2Voltage=global, Q3Current=global, Q3Voltage=global, VoltageSourceOutput=global
  wires:
  Logical Operator/1 -> Q3/1
  VoltageSourceOutput/1 -> [VoltageSourceOutput]  "VoltageSourceOutput"
  Q3Voltage/1 -> [Q3Voltage]  "Q3Voltage"
  Q2Voltage/1 -> [Q2Voltage]  "Q2Voltage"
  From9/1 -> Q2/1
  [SwitchingSignal2] -> Logical Operator/1
  L2Current/1 -> [L2Current]
  L2Voltage/1 -> [L2Voltage]
  L2Current1/1 -> [CCurrent]
  Q2Current/1 -> [Q2Current]  "Q2Current"
  Q3Current/1 -> [Q3Current]  "Q3Current"
  D2Current/1 -> [D2Current]  "D2Current"
  D3Current/1 -> [D3Current]  "D3Current"
  connections:
  " RLC 3"/RConn1 -- Out2/RConn1 -- In2/RConn1 -- Q3/RConn1 -- D3/LConn1 -- Q3Voltage/LConn2 -- VoltageSourceOutput/LConn2
  Q2Current/LConn1 -- In1/RConn1 -- D2Current/LConn1 -- Q2Voltage/LConn1
  L2Current1/LConn1 -- L2Current/RConn1 -- Out1/RConn1
  " RLC 2"/LConn1 -- L2Current/LConn1 -- L2Voltage/LConn1
  " RLC 7"/LConn1 -- VoltageSourceOutput/LConn1 -- L2Current1/RConn1
  Q2/RConn1 -- Q3Current/LConn1 -- Q2Voltage/LConn2 -- Q3Voltage/LConn1 -- D3Current/LConn1 -- D2/LConn1 -- " RLC 4"/RConn1 -- L2Voltage/LConn2
  " RLC 3"/LConn1 -- " RLC 7"/RConn1
  " RLC 2"/RConn1 -- " RLC 4"/LConn1
  Q2Current/RConn1 -- Q2/LConn1
  Q3Current/RConn1 -- Q3/LConn1
  D2Current/RConn1 -- D2/RConn1
  D3Current/RConn1 -- D3/RConn1

== system powersupply_1jan_old_top/PM0 ==
  Vin : Inport
  Iin : Inport  Port=2
  Product : Product
  Transfer Fcn : TransferFcn  Numerator=[2*pi*frq_dc]  Denominator=[1 2*pi*frq_dc]
  Ptrans : Outport
  Pavg : Outport  Port=2
  wires:
  Transfer Fcn/1 -> Pavg/1
  Iin/1 -> Product/2
  Product/1 -> Ptrans/1, Transfer Fcn/1
  Vin/1 -> Product/1

== system powersupply_1jan_old_top/Power Measurement1 ==
  Vin : Inport
  Iin : Inport  Port=2
  Product : Product
  Transfer Fcn : TransferFcn  Numerator=[2*pi*frq_dc]  Denominator=[1 2*pi*frq_dc]
  Ptrans : Outport
  Pavg : Outport  Port=2
  wires:
  Vin/1 -> Product/1
  Product/1 -> Transfer Fcn/1, Ptrans/1
  Iin/1 -> Product/2
  Transfer Fcn/1 -> Pavg/1

== system powersupply_1jan_old_top/Power Measurement11 ==
  Vin : Inport
  Iin : Inport  Port=2
  Product : Product
  Transfer Fcn : TransferFcn  Numerator=[2*pi*frq_dc]  Denominator=[1 2*pi*frq_dc]
  Ptrans : Outport
  Pavg : Outport  Port=2
  wires:
  Transfer Fcn/1 -> Pavg/1
  Iin/1 -> Product/2
  Product/1 -> Ptrans/1, Transfer Fcn/1
  Vin/1 -> Product/1

== system powersupply_1jan_old_top/Power Measurement12 ==
  Vin : Inport
  Iin : Inport  Port=2
  Product : Product
  Transfer Fcn : TransferFcn  Numerator=[2*pi*frq_dc]  Denominator=[1 2*pi*frq_dc]
  Ptrans : Outport
  Pavg : Outport  Port=2
  wires:
  Vin/1 -> Product/1
  Product/1 -> Transfer Fcn/1, Ptrans/1
  Iin/1 -> Product/2
  Transfer Fcn/1 -> Pavg/1

== system powersupply_1jan_old_top/Power Measurement2 ==
  Vin : Inport
  Iin : Inport  Port=2
  Product : Product
  Transfer Fcn : TransferFcn  Numerator=[2*pi*frq_dc]  Denominator=[1 2*pi*frq_dc]
  Ptrans : Outport
  Pavg : Outport  Port=2
  wires:
  Vin/1 -> Product/1
  Product/1 -> Transfer Fcn/1, Ptrans/1
  Iin/1 -> Product/2
  Transfer Fcn/1 -> Pavg/1

== system powersupply_1jan_old_top/Power Measurement3 ==
  Vin : Inport
  Iin : Inport  Port=2
  Product : Product
  Sum : Sum  Inputs=|+-
  Transfer Fcn : TransferFcn  Numerator=[2*pi*frq_dc]  Denominator=[1 2*pi*frq_dc]
  Transfer Fcn1 : TransferFcn  Numerator=[2*pi*frq_dc]  Denominator=[1 0]
  Ptrans : Outport
  Pavg : Outport  Port=2
  PavgFB : Outport  Port=3
  wires:
  Vin/1 -> Product/1
  Product/1 -> Sum/1, Transfer Fcn/1, Ptrans/1
  Iin/1 -> Product/2
  Transfer Fcn/1 -> Pavg/1
  Sum/1 -> Transfer Fcn1/1
  Transfer Fcn1/1 -> Sum/2, PavgFB/1

== system powersupply_1jan_old_top/Power Measurement4 ==
  Vin : Inport
  Iin : Inport  Port=2
  Product : Product
  Transfer Fcn : TransferFcn  Numerator=[2*pi*frq_dc]  Denominator=[1 2*pi*frq_dc]
  Ptrans : Outport
  Pavg : Outport  Port=2
  wires:
  Transfer Fcn/1 -> Pavg/1
  Iin/1 -> Product/2
  Product/1 -> Ptrans/1, Transfer Fcn/1
  Vin/1 -> Product/1

== system powersupply_1jan_old_top/Power Measurement5 ==
  Vin : Inport
  Iin : Inport  Port=2
  Product : Product
  Transfer Fcn : TransferFcn  Numerator=[2*pi*frq_dc]  Denominator=[1 2*pi*frq_dc]
  Ptrans : Outport
  Pavg : Outport  Port=2
  wires:
  Transfer Fcn/1 -> Pavg/1
  Iin/1 -> Product/2
  Product/1 -> Ptrans/1, Transfer Fcn/1
  Vin/1 -> Product/1

== system powersupply_1jan_old_top/Power Measurement6 ==
  Vin : Inport
  Iin : Inport  Port=2
  Product : Product
  Transfer Fcn : TransferFcn  Numerator=[2*pi*frq_dc]  Denominator=[1 2*pi*frq_dc]
  Ptrans : Outport
  Pavg : Outport  Port=2
  wires:
  Transfer Fcn/1 -> Pavg/1
  Iin/1 -> Product/2
  Product/1 -> Ptrans/1, Transfer Fcn/1
  Vin/1 -> Product/1

== system powersupply_1jan_old_top/Power Measurement7 ==
  Vin : Inport
  Iin : Inport  Port=2
  Product : Product
  Transfer Fcn : TransferFcn  Numerator=[2*pi*frq_dc]  Denominator=[1 2*pi*frq_dc]
  Ptrans : Outport
  Pavg : Outport  Port=2
  wires:
  Vin/1 -> Product/1
  Product/1 -> Transfer Fcn/1, Ptrans/1
  Iin/1 -> Product/2
  Transfer Fcn/1 -> Pavg/1

== system powersupply_1jan_old_top/Power Measurement8 ==
  Vin : Inport
  Iin : Inport  Port=2
  Product : Product
  Transfer Fcn : TransferFcn  Numerator=[2*pi*frq_dc]  Denominator=[1 2*pi*frq_dc]
  Ptrans : Outport
  Pavg : Outport  Port=2
  wires:
  Vin/1 -> Product/1
  Product/1 -> Transfer Fcn/1, Ptrans/1
  Iin/1 -> Product/2
  Transfer Fcn/1 -> Pavg/1

== system powersupply_1jan_old_top/Power Measurement9 ==
  Vin : Inport
  Iin : Inport  Port=2
  Product : Product
  Transfer Fcn : TransferFcn  Numerator=[2*pi*frq_dc]  Denominator=[1 2*pi*frq_dc]
  Ptrans : Outport
  Pavg : Outport  Port=2
  wires:
  Transfer Fcn/1 -> Pavg/1
  Iin/1 -> Product/2
  Product/1 -> Ptrans/1, Transfer Fcn/1
  Vin/1 -> Product/1

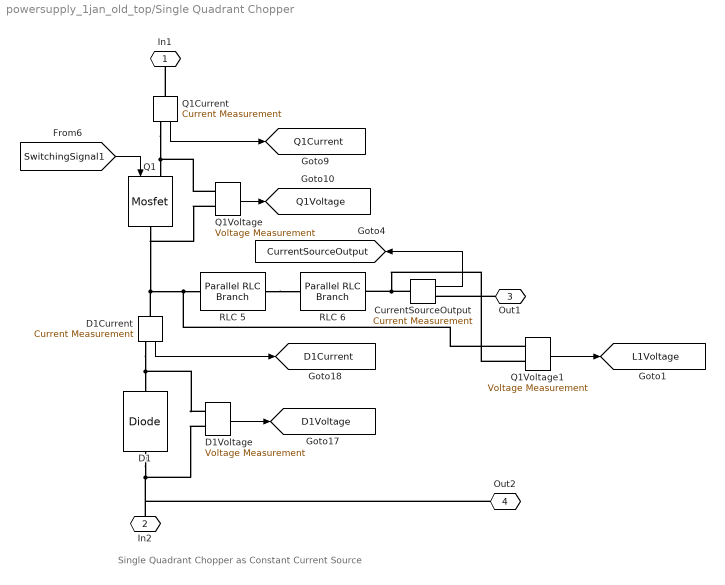
== system powersupply_1jan_old_top/Single Quadrant Chopper ==
  note: Single Quadrant Chopper as Constant Current Source
  " RLC 5" : powerlib/Elements/Parallel RLC Branch  LConnTagsString=a  RConnTagsString=__new0  BranchType=R  Resistance=rl1_val  Inductance=5e-6  SetiL0=off  InitialCurrent=0  Capacitance=0.3e-6  Setx0=off  InitialVoltage=0  Measurements=None
  " RLC 6" : powerlib/Elements/Parallel RLC Branch  LConnTagsString=a  RConnTagsString=__new0  BranchType=L  Resistance=50  Inductance=l1_val  SetiL0=off  InitialCurrent=100  Capacitance=0.3e-6  Setx0=off  InitialVoltage=0  Measurements=None
  CurrentSourceOutput : powerlib/Measurements/Current Measurement  PhasorSimulation=off  OutputType=Complex  PSBequivalent=0
  D1 : powerlib/Power Electronics/Diode  Ron=0.001  Lon=0  Vf=0.8  IC=0  UseSnubber=off  Rs=500  Cs=250e-9  Measurements=off
  D1Current : powerlib/Measurements/Current Measurement  PhasorSimulation=off  OutputType=Complex  PSBequivalent=0
  D1Voltage : powerlib/Measurements/Voltage Measurement  PhasorSimulation=off  OutputType=Complex  PSBequivalent=0
  Q1 : powerlib/Power Electronics/Mosfet  Ron=0.1  Lon=0  Rd=0.01  Vfd=0  IC=0  Rs=1e5  Cs=inf  Measurements=off
  Q1Current : powerlib/Measurements/Current Measurement  PhasorSimulation=off  OutputType=Complex  PSBequivalent=0
  Q1Voltage : powerlib/Measurements/Voltage Measurement  PhasorSimulation=off  OutputType=Complex  PSBequivalent=0
  Q1Voltage1 : powerlib/Measurements/Voltage Measurement  PhasorSimulation=off  OutputType=Complex  PSBequivalent=0
  In1 : PMIOPort  Port=1  Side=Left
  In2 : PMIOPort  Port=2  Side=Left
  Out1 : PMIOPort  Port=3  Side=Right
  Out2 : PMIOPort  Port=4  Side=Right
  tag scope: CurrentSourceOutput=global, D1Current=global, D1Voltage=global, L1Voltage=global, Q1Current=global, Q1Voltage=global
  wires:
  CurrentSourceOutput/1 -> [CurrentSourceOutput]
  [SwitchingSignal1] -> Q1/1
  Q1Current/1 -> [Q1Current]
  Q1Voltage/1 -> [Q1Voltage]
  D1Current/1 -> [D1Current]
  D1Voltage/1 -> [D1Voltage]
  Q1Voltage1/1 -> [L1Voltage]
  connections:
  Q1Voltage/LConn2 -- Q1/RConn1 -- D1Current/LConn1 -- Q1Voltage1/LConn1 -- " RLC 5"/LConn1
  Q1Current/LConn1 -- In1/RConn1
  " RLC 5"/RConn1 -- " RLC 6"/LConn1
  CurrentSourceOutput/LConn1 -- Q1Voltage1/LConn2 -- " RLC 6"/RConn1
  Q1Current/RConn1 -- Q1Voltage/LConn1 -- Q1/LConn1
  D1Current/RConn1 -- D1/RConn1 -- D1Voltage/LConn1
  D1Voltage/LConn2 -- In2/RConn1 -- Out2/RConn1 -- D1/LConn1
  Out1/RConn1 -- CurrentSourceOutput/RConn1

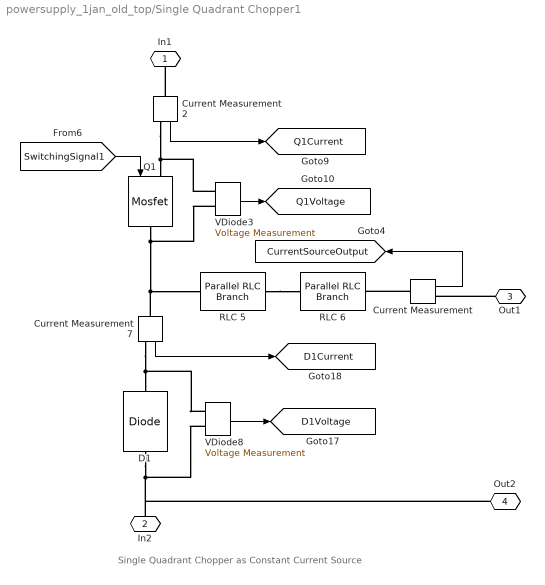
== system powersupply_1jan_old_top/Single Quadrant Chopper1 ==
  note: Single Quadrant Chopper as Constant Current Source
  " RLC 5" : powerlib/Elements/Parallel RLC Branch  LConnTagsString=a  RConnTagsString=__new0  BranchType=R  Resistance=rl1_val  Inductance=5e-6  SetiL0=off  InitialCurrent=0  Capacitance=0.3e-6  Setx0=off  InitialVoltage=0  Measurements=None
  " RLC 6" : powerlib/Elements/Parallel RLC Branch  LConnTagsString=a  RConnTagsString=__new0  BranchType=L  Resistance=50  Inductance=l1_val  SetiL0=off  InitialCurrent=100  Capacitance=0.3e-6  Setx0=off  InitialVoltage=0  Measurements=None
  Current Measurement2 : powerlib/Measurements/Current Measurement  PhasorSimulation=off  OutputType=Complex  PSBequivalent=0
  Current Measurement7 : powerlib/Measurements/Current Measurement  PhasorSimulation=off  OutputType=Complex  PSBequivalent=0
  Current Measurement : powerlib/Measurements/Current Measurement  PhasorSimulation=off  OutputType=Complex  PSBequivalent=0
  D1 : powerlib/Power Electronics/Diode  Ron=0.001  Lon=0  Vf=0.8  IC=0  UseSnubber=off  Rs=500  Cs=250e-9  Measurements=off
  Q1 : powerlib/Power Electronics/Mosfet  Ron=0.1  Lon=0  Rd=0.01  Vfd=0  IC=0  Rs=1e5  Cs=inf  Measurements=off
  VDiode3 : powerlib/Measurements/Voltage Measurement  PhasorSimulation=off  OutputType=Complex  PSBequivalent=0
  VDiode8 : powerlib/Measurements/Voltage Measurement  PhasorSimulation=off  OutputType=Complex  PSBequivalent=0
  In1 : PMIOPort  Port=1  Side=Left
  In2 : PMIOPort  Port=2  Side=Left
  Out1 : PMIOPort  Port=3  Side=Right
  Out2 : PMIOPort  Port=4  Side=Right
  tag scope: CurrentSourceOutput=global, D1Current=global, D1Voltage=global, Q1Current=global, Q1Voltage=global
  wires:
  Current Measurement/1 -> [CurrentSourceOutput]
  [SwitchingSignal1] -> Q1/1
  Current Measurement2/1 -> [Q1Current]
  VDiode3/1 -> [Q1Voltage]
  Current Measurement7/1 -> [D1Current]
  VDiode8/1 -> [D1Voltage]
  connections:
  VDiode3/LConn2 -- Q1/RConn1 -- Current Measurement7/LConn1 -- " RLC 5"/LConn1
  Current Measurement2/LConn1 -- In1/RConn1
  " RLC 5"/RConn1 -- " RLC 6"/LConn1
  Current Measurement/LConn1 -- " RLC 6"/RConn1
  Current Measurement2/RConn1 -- VDiode3/LConn1 -- Q1/LConn1
  Current Measurement7/RConn1 -- D1/RConn1 -- VDiode8/LConn1
  VDiode8/LConn2 -- In2/RConn1 -- Out2/RConn1 -- D1/LConn1
  Out1/RConn1 -- Current Measurement/RConn1

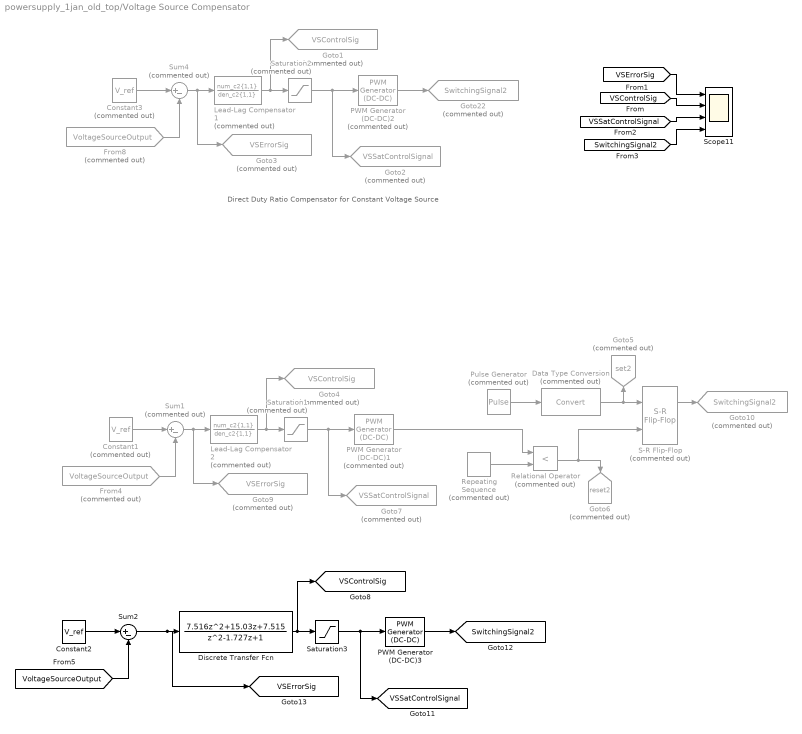
== system powersupply_1jan_old_top/Voltage Source Compensator ==
  note: Direct Duty Ratio Compensator for Constant Voltage Source
  Constant1 : Constant  Commented=on  Value=V_ref
  Constant2 : Constant  Value=V_ref
  Constant3 : Constant  Commented=on  Value=V_ref
  Data Type Conversion : DataTypeConversion  Commented=on
  Discrete Transfer Fcn : DiscreteTransferFcn  Numerator=[7.516 15.03 7.515]  Denominator=[1 -1.727 1]
  From4 : From  Commented=on  GotoTag=VoltageSourceOutput  TagVisibility=global
  From8 : From  Commented=on  GotoTag=VoltageSourceOutput  TagVisibility=global
  Goto1 : Goto  Commented=on  GotoTag=VSControlSig  TagVisibility=global
  Goto10 : Goto  Commented=on  GotoTag=SwitchingSignal2  TagVisibility=global
  Goto2 : Goto  Commented=on  GotoTag=VSSatControlSignal  TagVisibility=global
  Goto22 : Goto  Commented=on  GotoTag=SwitchingSignal2  TagVisibility=global
  Goto3 : Goto  Commented=on  GotoTag=VSErrorSig  TagVisibility=global
  Goto4 : Goto  Commented=on  GotoTag=VSControlSig  TagVisibility=global
  Goto5 : Goto  Commented=on  GotoTag=set2  TagVisibility=global
  Goto6 : Goto  Commented=on  GotoTag=reset2  TagVisibility=global
  Goto7 : Goto  Commented=on  GotoTag=VSSatControlSignal  TagVisibility=global
  Goto9 : Goto  Commented=on  GotoTag=VSErrorSig  TagVisibility=global
  Lead-Lag Compensator1 : TransferFcn  Commented=on  Numerator=num_c2{1,1}  Denominator=den_c2{1,1}
  Lead-Lag Compensator2 : TransferFcn  Commented=on  Numerator=num_c2{1,1}  Denominator=den_c2{1,1}
  PWM Generator (DC-DC)1 : powerlib_meascontrol/Pulse & Signal Generators/PWM Generator (DC-DC)  Commented=on  Fsw=f_sw  Ts=0
  PWM Generator (DC-DC)2 : powerlib_meascontrol/Pulse & Signal Generators/PWM Generator (DC-DC)  Commented=on  Fsw=f_sw  Ts=0
  PWM Generator (DC-DC)3 : powerlib_meascontrol/Pulse & Signal Generators/PWM Generator (DC-DC)  Fsw=f_sw  Ts=0
  Pulse Generator : DiscretePulseGenerator  Commented=on  PulseType=Time based  Period=1/f_sw  PulseWidth=5
  Relational Operator : RelationalOperator  Commented=on  Operator=<  OutDataTypeStr=boolean
  Repeating Sequence : simulink/Sources/Repeating Sequence  Commented=on  rep_seq_t=[0 1/f_sw]  rep_seq_y=[0 1]
  S-R Flip-Flop : simulink_extras/Flip Flops/S-R Flip-Flop  Commented=on  initial_condition=0
  Saturation1 : Saturate  Commented=on  UpperLimit=0.99  LowerLimit=0
  Saturation2 : Saturate  Commented=on  UpperLimit=0.99  LowerLimit=0
  Saturation3 : Saturate  UpperLimit=0.99  LowerLimit=0
  Scope11 : Scope  NumInputPorts=4
  Sum1 : Sum  Commented=on  Inputs=|+-
  Sum2 : Sum  Inputs=|+-
  Sum4 : Sum  Commented=on  Inputs=|+-
  tag scope: SwitchingSignal2=global, VSControlSig=global, VSErrorSig=global, VSSatControlSignal=global
  wires:
  Sum4/1 -> Lead-Lag Compensator1/1, Goto3/1
  Constant3/1 -> Sum4/1
  From8/1 -> Sum4/2
  Lead-Lag Compensator1/1 -> Goto1/1, Saturation2/1
  Saturation2/1 -> Goto2/1, PWM Generator (DC-DC)2/1
  PWM Generator (DC-DC)2/1 -> Goto22/1
  [VSErrorSig] -> Scope11/1
  [SwitchingSignal2] -> Scope11/4
  [VSSatControlSignal] -> Scope11/3
  [VSControlSig] -> Scope11/2
  Pulse Generator/1 -> Data Type Conversion/1
  Data Type Conversion/1 -> S-R Flip-Flop/1, Goto5/1
  Relational Operator/1 -> S-R Flip-Flop/2, Goto6/1
  S-R Flip-Flop/1 -> Goto10/1
  PWM Generator (DC-DC)1/1 -> Relational Operator/1
  Repeating Sequence/1 -> Relational Operator/2
  Sum1/1 -> Lead-Lag Compensator2/1, Goto9/1
  Constant1/1 -> Sum1/1
  From4/1 -> Sum1/2
  Lead-Lag Compensator2/1 -> Goto4/1, Saturation1/1
  Saturation1/1 -> Goto7/1, PWM Generator (DC-DC)1/1
  Sum2/1 -> [VSErrorSig], Discrete Transfer Fcn/1
  Constant2/1 -> Sum2/1
  [VoltageSourceOutput] -> Sum2/2
  Discrete Transfer Fcn/1 -> Saturation3/1, [VSControlSig]
  Saturation3/1 -> [VSSatControlSignal], PWM Generator (DC-DC)3/1
  PWM Generator (DC-DC)3/1 -> [SwitchingSignal2]
